simulink model "cm_ldpc_decode_qpsk_signal"  (R2020a)
settings: Solver=VariableStepAuto  StartTime=0.0  StopTime=0  RelTol=1e-3
InitFcn:
  | snr = 1.0;
undefined symbols (not defined in the file or in its folder): dvbs2ldpc
libraries: commblkcod2 x2, commdigbbndpm3 x2, commchan3 x1, commsink2 x1
settings Model: Creator=The MathWorks, Inc.  LastModifiedBy=The MathWorks, Inc.
settings DataIOCC: ReturnWorkspaceOutputs=off
settings DebuggingCC: ArithmeticOperatorsInVariantConditions=warning
settings SFSimCC: SimUseLocalCustomCode=off  CustomCodeUndefinedFunction=UseInterfaceOnly
settings RTWCC: RTWUseLocalCustomCode=off
settings CodeAppCC: StateflowObjectComments=on
settings GRTTargetCC: TargetLangStandard=C89/C90 (ANSI)
settings ConfigComp: CovMetricSettings=dsw  CovHtmlReporting=on  CovSaveCumulativeToWorkspaceVar=on  CovSaveSingleToWorkspaceVar=on  CovShowResultsExplorer=off  CovExternalEMLEnable=off

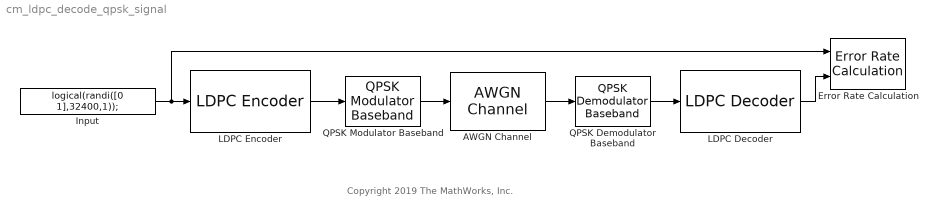
== system cm_ldpc_decode_qpsk_signal ==
  note: Copyright 2019 The MathWorks, Inc.
  AWGN Channel : commchan3/AWGN Channel  InputProcessing=Columns as channels (frame based)  seed=67  noiseMode="Signal to noise ratio  (SNR)"  EbNodB=snr  EsNodB=10  SNRdB=snr  bitsPerSym=1  Ps=1  Tsym=1  variance=1
  Error Rate Calculation : commsink2/Error Rate Calculation  N=0  st_delay=0  cp_mode=Entire frame  subframe=[]  PMode=Workspace  WsName=ErrorVec  RsMode2=off  stop=off  numErr=100  maxBits=1e6
  Input : Constant  Value=logical(randi([0 1],32400,1));  VectorParams1D=off  OutDataTypeStr=boolean  SampleTime=1
  LDPC Decoder : commblkcod2/LDPC Decoder  ParityCheckMat=dvbs2ldpc(1/2)  OutputFmt=Information part  DecisionType=Hard decision  OutputDataType=boolean  NumIter=50  DoParityCheck=off  OutputNumIter=off  OutputFinalChecks=off
      settings: SourceProductBaseCode=CM
  LDPC Encoder : commblkcod2/LDPC Encoder  ParityCheckMat=dvbs2ldpc(1/2)
      settings: SourceProductBaseCode=CM
  QPSK Demodulator Baseband : commdigbbndpm3/QPSK Demodulator Baseband  OutType=Bit  DecType=Approximate log-likelihood ratio  VarSource=Dialog  Variance=1/10^(snr/10)  Dec=Gray  Ph=pi/4  outDtype1=Inherit via internal rule  outDtype2=Inherit via internal rule  derotateFactorWordLen=16  derotateFactorDataTypeStr=Inherit: Same word length as input  derotateFactorLastDataTypeStr=Inherit: Same word length as input
  QPSK Modulator Baseband : commdigbbndpm3/QPSK Modulator Baseband  InType=Bit  Enc=Gray  Ph=pi/4  outDtype=double  outWordLen=16  outUDDataType=sfix(16)  outFracLenMode=Best precision  outFracLen=15  outDataTypeStr=double  outLastDataTypeStr=double
  wires:
  Input/1 -> Error Rate Calculation/1, LDPC Encoder/1
  LDPC Encoder/1 -> QPSK Modulator Baseband/1
  QPSK Modulator Baseband/1 -> AWGN Channel/1
  AWGN Channel/1 -> QPSK Demodulator Baseband/1
  QPSK Demodulator Baseband/1 -> LDPC Decoder/1
  LDPC Decoder/1 -> Error Rate Calculation/2
